simulink model "ruehrkesselReaktor"  (R2021b)
settings: Solver=VariableStepAuto  StartTime=0.0  StopTime=3600  RelTol=1e-3
values from neighbouring files (symbols this model uses):
  k = ((1/alpha1)+(s/Waermeleitfaeigkeit)+(1/alpha2))^(-1)    (= 653.590289794)    [auslegungGBS418M_WT.m]    (also in auslegungTL3_WT.m = 310.873015337)
undefined symbols (not defined in the file or in its folder): Aw, c1_0, c2_0, c3_0, cp, deltaRH, kw, m, V
settings Model: Creator=philippsum  LastModifiedBy=philippsum

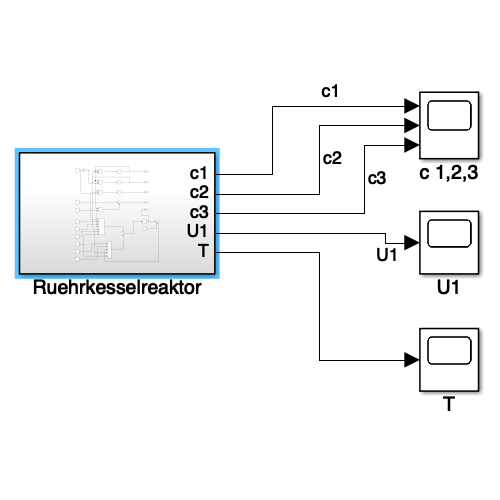
[thumbnail: Simulink's stored preview of the top-level diagram]
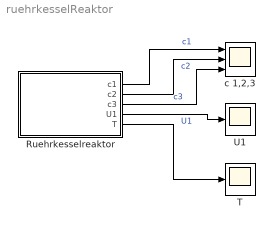
== system ruehrkesselReaktor ==
  Ruehrkesselreaktor : Subsystem
  T : Scope
  U1 : Scope
  c 1,2,3 : Scope  NumInputPorts=3
  wires:
  Ruehrkesselreaktor/1(c1) -> c 1,2,3/1  "c1"
  Ruehrkesselreaktor/2(c2) -> c 1,2,3/2  "c2"
  Ruehrkesselreaktor/3(c3) -> c 1,2,3/3  "c3"
  Ruehrkesselreaktor/4(U1) -> U1/1  "U1"
  Ruehrkesselreaktor/5(T) -> T/1

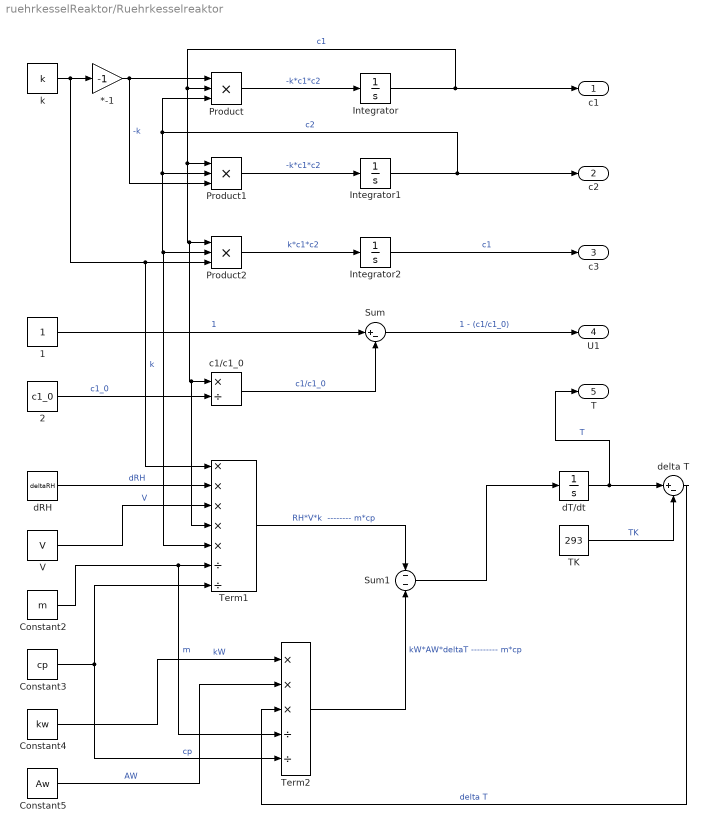
== system ruehrkesselReaktor/Ruehrkesselreaktor ==
  *-1 : Gain  Gain=-1
  1 : Constant
  2 : Constant  Value=c1_0  VectorParams1D=off
  Constant2 : Constant  Value=m
  Constant3 : Constant  Value=cp
  Constant4 : Constant  Value=kw
  Constant5 : Constant  Value=Aw
  Integrator : Integrator  InitialCondition=c1_0
  Integrator1 : Integrator  InitialCondition=c2_0
  Integrator2 : Integrator  InitialCondition=c3_0
  Product : Product  Inputs=3
  Product1 : Product  Inputs=3
  Product2 : Product  Inputs=3
  Sum : Sum  Inputs=|+-
  Sum1 : Sum  Inputs=--
  TK : Constant  Value=293
  Term1 : Product  Inputs=*****//
  Term2 : Product  Inputs=***//
  V : Constant  Value=V
  c1/c1_0 : Product  Inputs=*/
  dRH : Constant  Value=deltaRH
  dT/dt : Integrator
  delta T : Sum  Inputs=|+-
  k : Constant  Value=k
  c1 : Outport
  c2 : Outport  Port=2
  c3 : Outport  Port=3
  U1 : Outport  Port=4
  T : Outport  Port=5
  wires:
  Integrator/1 -> Term1/4, c1/c1_0/1, Product2/1, Product1/1, Product/2, c1/1  "c1"
  k/1 -> Term1/1, Product2/3, *-1/1  "k"
  *-1/1 -> Product1/3, Product/1  "-k"
  Integrator1/1 -> c2/1, Term1/5, Product2/2, Product1/2, Product/3  "c2"
  Product/1 -> Integrator/1  "-k*c1*c2"
  Product1/1 -> Integrator1/1  "-k*c1*c2"
  Product2/1 -> Integrator2/1  "k*c1*c2"
  Integrator2/1 -> c3/1  "c1"
  1/1 -> Sum/1  "1"
  2/1 -> c1/c1_0/2  "c1_0"
  c1/c1_0/1 -> Sum/2  "c1/c1_0"
  Sum/1 -> U1/1  "1 - (c1/c1_0)"
  dT/dt/1 -> T/1, delta T/1  "T"
  TK/1 -> delta T/2  "TK"
  dRH/1 -> Term1/2  "dRH"
  V/1 -> Term1/3  "V"
  Constant2/1 -> Term2/4, Term1/6  "m"
  Constant3/1 -> Term2/5, Term1/7  "cp"
  Constant4/1 -> Term2/1  "kW"
  Constant5/1 -> Term2/2  "AW"
  delta T/1 -> Term2/3  "delta T"
  Term1/1 -> Sum1/1  "RH*V*k  -------- m*cp"
  Term2/1 -> Sum1/2  "kW*AW*deltaT --------- m*cp"
  Sum1/1 -> dT/dt/1
